simulink model "FIR_filter1"  (R2020b)
settings: Solver=FixedStepAuto  StartTime=0.0  StopTime=10.0  FixedStep=0.2  RelTol=1e-3
model workspace (MAT data in the model file):
  b0 = 1
  b1 = 2
  b2 = -3
  b3 = -4
  b4 = 5
settings Model: Creator=rutvi  LastModifiedBy=rutvi
settings DataIOCC: SaveOutput=off  SaveTime=off

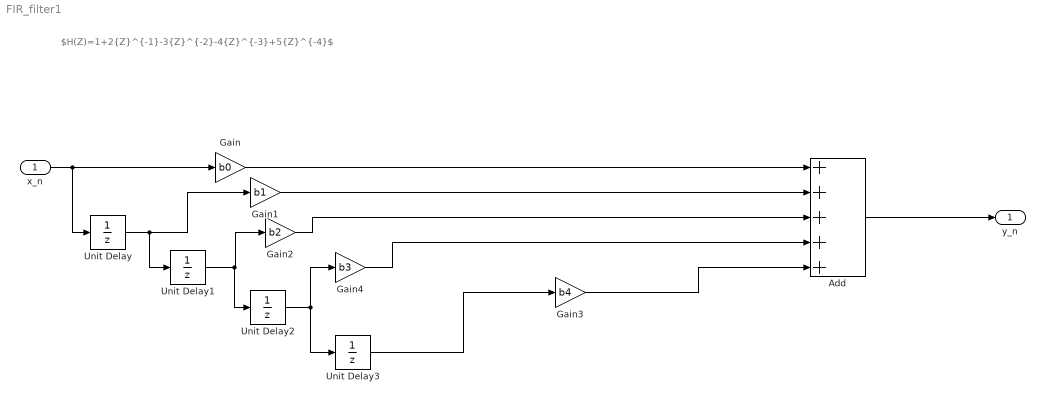
== system FIR_filter1 ==
  note: $H(Z)=1+2{Z}^{-1}-3{Z}^{-2}-4{Z}^{-3}+5{Z}^{-4}$
  x_n : Inport  OutDataTypeStr=double  PortDimensions=1
  Add : Sum  Inputs=+++++
  Gain : Gain  Gain=b0
  Gain1 : Gain  Gain=b1
  Gain2 : Gain  Gain=b2
  Gain3 : Gain  Gain=b4
  Gain4 : Gain  Gain=b3
  Unit Delay{,1..3} (4 alike) : UnitDelay  SampleTime=-1  HasFrameUpgradeWarning=on
  y_n : Outport  OutDataTypeStr=double  PortDimensions=1  SampleTime=[0.20000000000000001,0]
  wires:
  x_n/1 -> Unit Delay/1, Gain/1
  Add/1 -> y_n/1
  Gain/1 -> Add/1
  Unit Delay/1 -> Gain1/1, Unit Delay1/1
  Gain1/1 -> Add/2
  Unit Delay1/1 -> Gain2/1, Unit Delay2/1
  Gain2/1 -> Add/3
  Unit Delay2/1 -> Gain4/1, Unit Delay3/1
  Gain4/1 -> Add/4
  Gain3/1 -> Add/5
  Unit Delay3/1 -> Gain3/1
